simulink model "steering_wheel_dynamics"  (R2022b)
settings: Solver=VariableStepAuto  StartTime=0.0  StopTime=10  RelTol=1e-3
undefined symbols (not defined in the file): Bm1, Bsc, Im1, Isw, Ke, Ksc, Kt, L1, R1, Tfrc, Vs1
libraries: simulink_extras x1
settings Model: Creator=Timothy  LastModifiedBy=Timothy

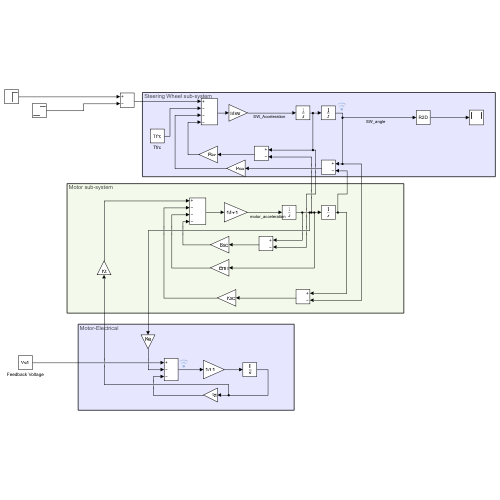
[thumbnail: Simulink's stored preview of the top-level diagram]
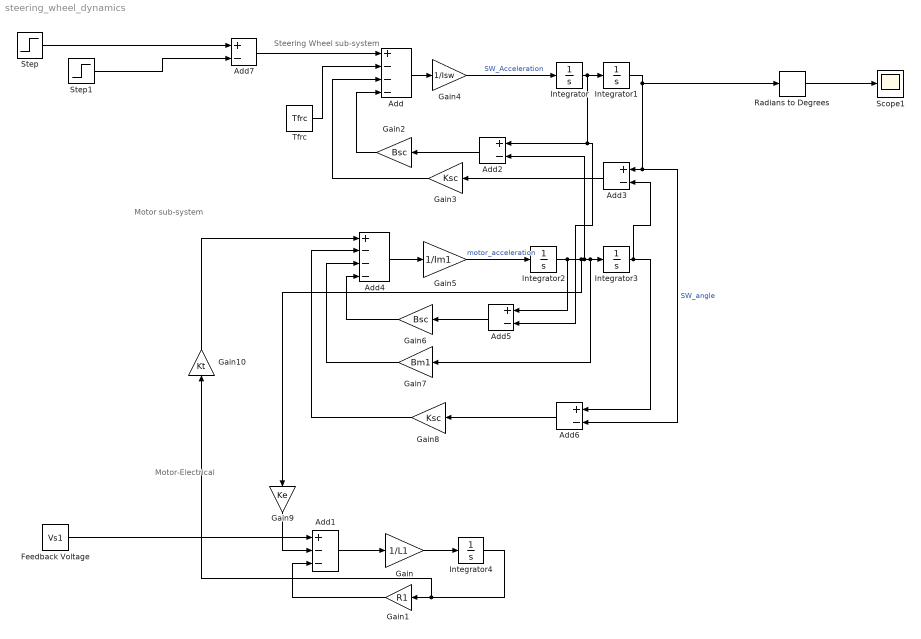
== system steering_wheel_dynamics ==
  note: Motor-Electrical
  note: Steering Wheel sub-system
  note: Motor sub-system
  Add : Sum  Inputs=+---
  Add1 : Sum  Inputs=+--
  Add{2..3,5..7} (5 alike) : Sum  Inputs=+-
  Add4 : Sum  Inputs=+---
  Feedback Voltage : Constant  Value=Vs1
  Gain : Gain  Gain=1/L1
  Gain1 : Gain  Gain=R1
  Gain10 : Gain  Gain=Kt
  Gain2 : Gain  Gain=Bsc
  Gain3 : Gain  Gain=Ksc
  Gain4 : Gain  Gain=1/Isw
  Gain5 : Gain  Gain=1/Im1
  Gain6 : Gain  Gain=Bsc
  Gain7 : Gain  Gain=Bm1
  Gain8 : Gain  Gain=Ksc
  Gain9 : Gain  Gain=Ke
  Integrator{,1..4} (5 alike) : Integrator
  Radians to Degrees : simulink_extras/Transformations/Radians to Degrees
  Scope1 : Scope
  Step : Step  SampleTime=0
  Step1 : Step  Time=2  SampleTime=0
  Tfrc : Constant  Value=Tfrc
  wires:
  Add6/1 -> Gain8/1
  Integrator3/1 -> Add3/2, Add6/1
  Add2/1 -> Gain2/1
  Add4/1 -> Gain5/1
  Integrator2/1 -> Gain9/1, Add2/2, Gain7/1, Integrator3/1, Add5/1
  Gain3/1 -> Add/3
  Gain7/1 -> Add4/3
  Add3/1 -> Gain3/1
  Radians to Degrees/1 -> Scope1/1
  Gain4/1 -> Integrator/1  "SW_Acceleration"
  Add/1 -> Gain4/1
  Gain6/1 -> Add4/4
  Add5/1 -> Gain6/1
  Gain2/1 -> Add/4
  Integrator4/1 -> Gain1/1, Gain10/1
  Integrator1/1 -> Add6/2, Add3/1, Radians to Degrees/1  "SW_angle"
  Integrator/1 -> Integrator1/1, Add2/1, Add5/2
  Gain8/1 -> Add4/2
  Gain5/1 -> Integrator2/1  "motor_acceleration"
  Tfrc/1 -> Add/2
  Add7/1 -> Add/1
  Add1/1 -> Gain/1
  Feedback Voltage/1 -> Add1/1
  Gain/1 -> Integrator4/1
  Gain1/1 -> Add1/3
  Gain9/1 -> Add1/2
  Gain10/1 -> Add4/1
  Step/1 -> Add7/1
  Step1/1 -> Add7/2
